simulink model "project2_roomba_wifitest"  (R2017a)
settings: Solver=VariableStepAuto  StartTime=0.0  StopTime=Inf  RelTol=1e-3
libraries: martin_sean_RoombaLib x5, realtime_pacer_lib x1
settings Model: Creator=bai  LastModifiedBy=Lab

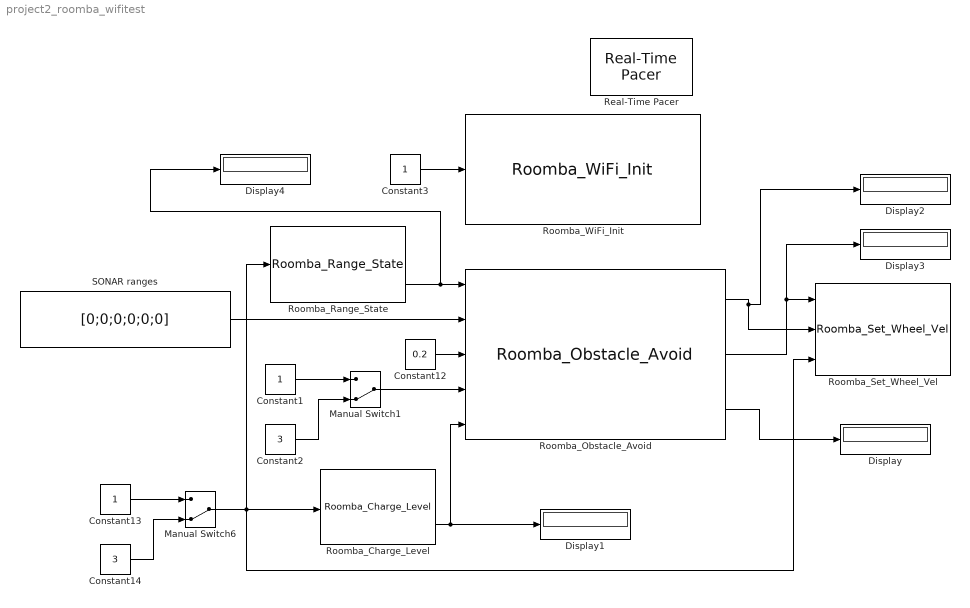
== system project2_roomba_wifitest ==
  Constant1 : Constant
  Constant12 : Constant  Value=0.2
  Constant13 : Constant
  Constant14 : Constant  Value=3
  Constant2 : Constant  Value=3
  Constant3 : Constant
  Display{,1..4} (5 alike) : Display
  Manual Switch1 : ManualSwitch  CurrentSetting=0
  Manual Switch6 : ManualSwitch  CurrentSetting=0
  Real-Time Pacer : realtime_pacer_lib/Real-Time Pacer  simTimePerRealTime=1
  Roomba_Charge_Level : martin_sean_RoombaLib/Roomba_Charge_Level  Description=Returns the battery charge level on the Roomba as a percentage. Updates every 100 seconds.
  Roomba_Obstacle_Avoid : martin_sean_RoombaLib/Roomba_Obstacle_Avoid
  Roomba_Range_State : martin_sean_RoombaLib/Roomba_Range_State  Description=|
      | Returns [1x6] array containing the state of the six IR sensors on the front of the Roomba. A 
      | '1' indicates there is an object ahead and a '0' indicates no object.
  Roomba_Set_Wheel_Vel : martin_sean_RoombaLib/Roomba_Set_Wheel_Vel  Description=|
      | Sets the right and left wheel velocities on the Roomba. The values are in meters/sec between 
      | [-0.5, 0.5]. Negative velocity is backwards.
  Roomba_WiFi_Init : martin_sean_RoombaLib/Roomba_WiFi_Init  Description=|  Priority=-1000
      | Initializes a WiFi connection to the Roomba. The RooWiFi module is used. Takes the mode as an
      | input. For instance, Mode = 1 will set up a connection to the Roomba over RooWiFi on 10.0.0.1
      | and place it in 'full' mode.
      | 
      | A 0 is returned after successful initialization.
      | 
      | RooWiFi documentation:
      | http://www.roowifi.com/wp-content/uploads/RwRemote_User_Guide_v2_rev15.pdf
  SONAR ranges : Constant  Value=[0;0;0;0;0;0]
  wires:
  Constant13/1 -> Manual Switch6/1
  Constant14/1 -> Manual Switch6/2
  SONAR ranges/1 -> Roomba_Obstacle_Avoid/2
  Constant12/1 -> Roomba_Obstacle_Avoid/3
  Roomba_Charge_Level/2 -> Roomba_Obstacle_Avoid/5, Display1/1
  Manual Switch6/1 -> Roomba_Set_Wheel_Vel/3, Roomba_Range_State/1, Roomba_Charge_Level/1
  Constant1/1 -> Manual Switch1/1
  Constant2/1 -> Manual Switch1/2
  Manual Switch1/1 -> Roomba_Obstacle_Avoid/4
  Roomba_Obstacle_Avoid/2 -> Display3/1, Roomba_Set_Wheel_Vel/1
  Roomba_Obstacle_Avoid/1 -> Display2/1, Roomba_Set_Wheel_Vel/2
  Roomba_Obstacle_Avoid/3 -> Display/1
  Constant3/1 -> Roomba_WiFi_Init/1
  Roomba_Range_State/2 -> Roomba_Obstacle_Avoid/1, Display4/1
